simulink model "first_version"  (R2016a)
settings: Solver=VariableStepAuto  StartTime=0.0  StopTime=0.12  RelTol=1e-3
libraries: powerlib x22, powerlib_meascontrol x3
settings Model: Creator=hakan  LastModifiedBy=hakan
settings DebuggingCC: UnconnectedInputMsg=none  UnconnectedOutputMsg=none  UnconnectedLineMsg=none

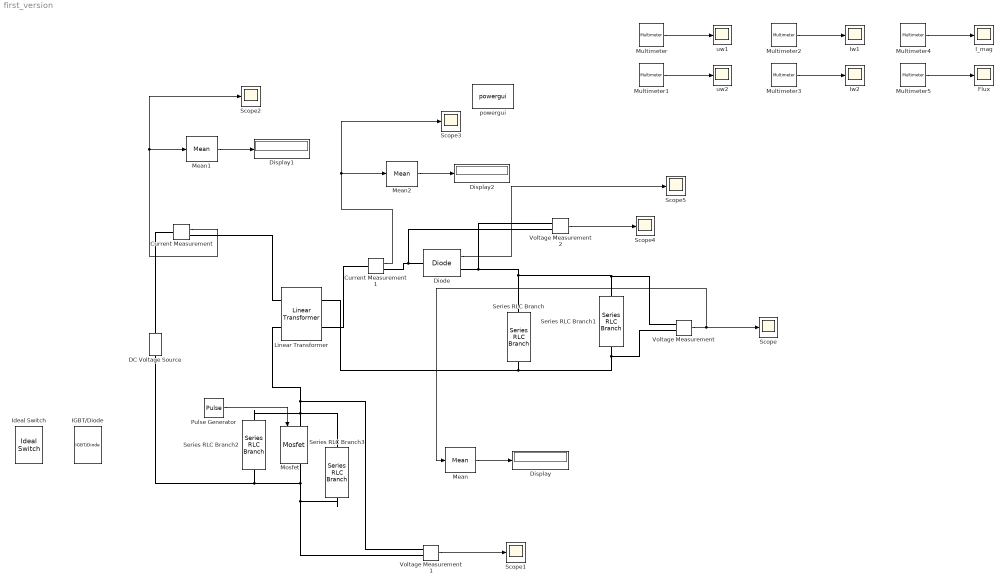
== system first_version ==
  Current Measurement : powerlib/Measurements/Current Measurement  PhasorSimulation=off  OutputType=Complex  PSBequivalent=0
  Current Measurement1 : powerlib/Measurements/Current Measurement  PhasorSimulation=off  OutputType=Complex  PSBequivalent=0
  DC Voltage Source : powerlib/Electrical Sources/DC Voltage Source  Amplitude=24  Measurements=None
  Diode : powerlib/Power Electronics/Diode  Ron=0.001  Lon=0  Vf=0.8  IC=0  UseSnubber=off  Rs=500  Cs=250e-9  Measurements=on
  Display : Display
  Display1 : Display
  Display2 : Display
  Flux : Scope
  IGBT/Diode : powerlib/Power Electronics/IGBT//Diode  Ron=1e-3  Rs=1e5  Cs=inf  Measurements=on
  I_mag : Scope
  Ideal Switch : powerlib/Power Electronics/Ideal Switch  Ron=0.001  Lon=0  IC=0  Rs=1e5  Cs=inf  Measurements=on
  "Iw1 " : Scope
  Iw2 : Scope
  Linear Transformer : powerlib/Elements/Linear Transformer  UNITS=SI  NominalPower=[ 100 50e3 ]  winding1=[30 0.03 2.2919e-06]  winding2=[15 0.015 5.7297e-07]  ThreeWindings=off  winding3=[3.15e+05 1.9845e+06 252.67]  RmLm=[4500 250e-6]  Measurements=All voltages and currents  DataType=on
  Mean : powerlib_meascontrol/Measurements/Mean  Freq=60  Vinit=0  Ts=0
  Mean1 : powerlib_meascontrol/Measurements/Mean  Freq=60  Vinit=0  Ts=0
  Mean2 : powerlib_meascontrol/Measurements/Mean  Freq=10000  Vinit=0  Ts=0
  Mosfet : powerlib/Power Electronics/Mosfet  Ron=0.16  Lon=0  Rd=0.01  Vfd=0  IC=0  Rs=1e5  Cs=inf  Measurements=on
  Multimeter : powerlib/Measurements/Multimeter  PhasorSimulation=off  OutputType=Complex  sel=1  L=7  Gain=1  yselected={'Uw1: Linear Transformer'};  PSBOutputType=1  PSBequivalent=0  AxesSetting=[0,0.1,-100,100]  Display=0  SavedBlockNames=-11
  Multimeter1 : powerlib/Measurements/Multimeter  PhasorSimulation=off  OutputType=Complex  sel=2  L=7  Gain=1  yselected={'Uw2: Linear Transformer'};  PSBOutputType=1  PSBequivalent=0  AxesSetting=[0,0.1,-100,100]  Display=0  SavedBlockNames=-11
  Multimeter2 : powerlib/Measurements/Multimeter  PhasorSimulation=off  OutputType=Complex  sel=3  L=7  Gain=1  yselected={'Iw1: Linear Transformer'};  PSBOutputType=1  PSBequivalent=0  AxesSetting=[0,0.1,-100,100]  Display=0  SavedBlockNames=-11
  Multimeter3 : powerlib/Measurements/Multimeter  PhasorSimulation=off  OutputType=Complex  sel=4  L=7  Gain=1  yselected={'Iw2: Linear Transformer'};  PSBOutputType=1  PSBequivalent=0  AxesSetting=[0,0.1,-100,100]  Display=0  SavedBlockNames=-11
  Multimeter4 : powerlib/Measurements/Multimeter  PhasorSimulation=off  OutputType=Complex  sel=6  L=7  Gain=1  yselected={'Imag: Linear Transformer'};  PSBOutputType=1  PSBequivalent=0  AxesSetting=[0,0.1,-100,100]  Display=0  SavedBlockNames=-11
  Multimeter5 : powerlib/Measurements/Multimeter  PhasorSimulation=off  OutputType=Complex  sel=7  L=7  Gain=1  yselected={'Flux: Linear Transformer'};  PSBOutputType=1  PSBequivalent=0  AxesSetting=[0,0.1,-100,100]  Display=0  SavedBlockNames=-11
  Pulse Generator : DiscretePulseGenerator  PulseType=Time based  Period=1/10000  PulseWidth=55
  Scope{,1..5} (6 alike) : Scope
  Series RLC Branch : powerlib/Elements/Series RLC Branch  LConnTagsString=__new0  RConnTagsString=__new0  BranchType=C  Resistance=1  Inductance=1e-3  SetiL0=off  InitialCurrent=0  Capacitance=1000e-6  Setx0=off  InitialVoltage=0  Measurements=None
  Series RLC Branch1 : powerlib/Elements/Series RLC Branch  LConnTagsString=__new0  RConnTagsString=__new0  BranchType=R  Resistance=1.8  Inductance=1e-3  SetiL0=off  InitialCurrent=0  Capacitance=1e-6  Setx0=off  InitialVoltage=0  Measurements=None
  Series RLC Branch2 : powerlib/Elements/Series RLC Branch  LConnTagsString=__new0  RConnTagsString=__new0  BranchType=C  Resistance=70  Inductance=1e-3  SetiL0=off  InitialCurrent=0  Capacitance=930e-12  Setx0=off  InitialVoltage=0  Measurements=None
  Series RLC Branch3 : powerlib/Elements/Series RLC Branch  LConnTagsString=__new0  RConnTagsString=__new0  BranchType=RC  Resistance=3.3  Inductance=1e-3  SetiL0=off  InitialCurrent=0  Capacitance=2e-6  Setx0=off  InitialVoltage=0  Measurements=None
  Voltage Measurement : powerlib/Measurements/Voltage Measurement  PhasorSimulation=off  OutputType=Complex  PSBequivalent=0
  Voltage Measurement1 : powerlib/Measurements/Voltage Measurement  PhasorSimulation=off  OutputType=Complex  PSBequivalent=0
  Voltage Measurement2 : powerlib/Measurements/Voltage Measurement  PhasorSimulation=off  OutputType=Complex  PSBequivalent=0
  powergui : powerlib/powergui  Priority=1  SimulationMode=Continuous  SolverType=Tustin/Backward Euler (TBE)  SampleTime=50e-6  frequency=60  SPID=off  DisableSnubberDevices=off  DisableRonSwitches=off  DisableVfSwitches=off  SwTol=0  DisplayEquations=off  Interpol=off  ExternalGateDelay=off  methode=off  Ts=10  FunctionMessages=off  echomessages=off  HookPort=off  EnableUseOfTLC=off  x0status=blocks  frequencyindice=0  Pbase=100e6  ErrMax=1e-4  Iterations=50  UnitsV=kV  UnitsW=MW  buscounter=0  RestoreLinks=warning  ResistiveCurrentMeasurement=off  Frange=[0:2:500]  Ylog=off  Xlog=on  ShowGrid=off  save=off  variable=ZData  structure=0  ZoomFFT=off  StartTime=0.0  cycles=1  DisplayStyle=1  fundamental=60  FreqAxis=off  MaxFrequency=1000  frequencyindicesteady=1  RmsSteady=1  display=off
  uw1 : Scope
  uw2 : Scope
  wires:
  Pulse Generator/1 -> Mosfet/1
  Voltage Measurement/1 -> Mean/1, Scope/1
  Mean/1 -> Display/1
  Multimeter/1 -> uw1/1
  Multimeter1/1 -> uw2/1
  Multimeter2/1 -> "Iw1 "/1
  Multimeter3/1 -> Iw2/1
  Multimeter4/1 -> I_mag/1
  Multimeter5/1 -> Flux/1
  Voltage Measurement1/1 -> Scope1/1
  Mean1/1 -> Display1/1
  Current Measurement/1 -> Scope2/1, Mean1/1
  Mean2/1 -> Display2/1
  Current Measurement1/1 -> Mean2/1, Scope3/1
  Voltage Measurement2/1 -> Scope4/1
  Diode/1 -> Scope5/1
  connections:
  DC Voltage Source/RConn1 -- Current Measurement/LConn1
  Linear Transformer/LConn2 -- Series RLC Branch3/LConn1 -- Mosfet/LConn1 -- Series RLC Branch2/LConn1 -- Voltage Measurement1/LConn1
  DC Voltage Source/LConn1 -- Series RLC Branch3/RConn1 -- Voltage Measurement1/LConn2 -- Mosfet/RConn1 -- Series RLC Branch2/RConn1
  Diode/RConn1 -- Voltage Measurement2/LConn1 -- Voltage Measurement/LConn1 -- Series RLC Branch1/LConn1 -- Series RLC Branch/LConn1
  Voltage Measurement/LConn2 -- Series RLC Branch1/RConn1 -- Linear Transformer/RConn1 -- Series RLC Branch/RConn1
  Current Measurement/RConn1 -- Linear Transformer/LConn1
  Linear Transformer/RConn2 -- Current Measurement1/LConn1
  Current Measurement1/RConn1 -- Voltage Measurement2/LConn2 -- Diode/LConn1
